simulink model "CRA_Assignment3"  (R2022b)
settings: Solver=VariableStepAuto  StartTime=0.0  StopTime=100  RelTol=1e-3
settings Model: Creator=lerio  LastModifiedBy=lerio

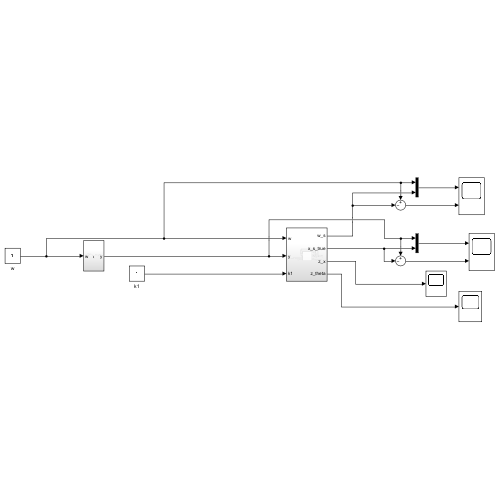
[thumbnail: Simulink's stored preview of the top-level diagram]
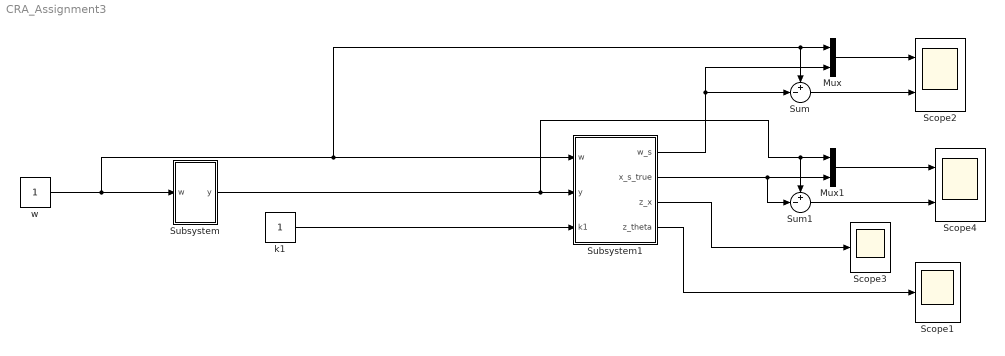
== system CRA_Assignment3 ==
  Mux : Mux  Inputs=2
  Mux1 : Mux  Inputs=2
  Scope1 : Scope
  Scope2 : Scope  NumInputPorts=2
  Scope3 : Scope
  Scope4 : Scope  NumInputPorts=2
  Subsystem : Subsystem
  Subsystem1 : Subsystem
  Sum : Sum  Inputs=+-|
  Sum1 : Sum  Inputs=+-|
  k1 : Constant
  w : Constant
  wires:
  w/1 -> Sum/1, Mux/1, Subsystem1/1(w), Subsystem/1(w)
  Subsystem/1(y) -> Sum1/1, Mux1/1, Subsystem1/2(y)
  k1/1 -> Subsystem1/3(k1)
  Mux/1 -> Scope2/1
  Subsystem1/1(w_s) -> Sum/2, Mux/2
  Sum/1 -> Scope2/2
  Mux1/1 -> Scope4/1
  Sum1/1 -> Scope4/2
  Subsystem1/2(x_s_true) -> Sum1/2, Mux1/2
  Subsystem1/3(z_x) -> Scope3/1
  Subsystem1/4(z_theta) -> Scope1/1

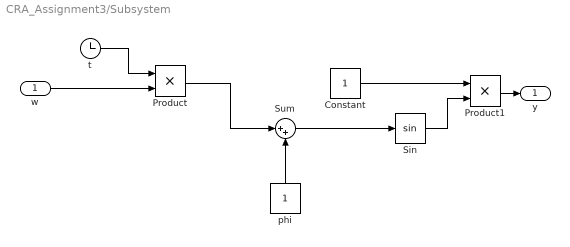
== system CRA_Assignment3/Subsystem ==
  w : Inport
  Constant : Constant
  Product : Product
  Product1 : Product
  Sin : Trigonometry
  Sum : Sum  Inputs=|++
  phi : Constant
  t : Clock
  y : Outport
  wires:
  Product1/1 -> y/1
  Constant/1 -> Product1/1
  Sin/1 -> Product1/2
  t/1 -> Product/1
  phi/1 -> Sum/2
  Product/1 -> Sum/1
  w/1 -> Product/2
  Sum/1 -> Sin/1

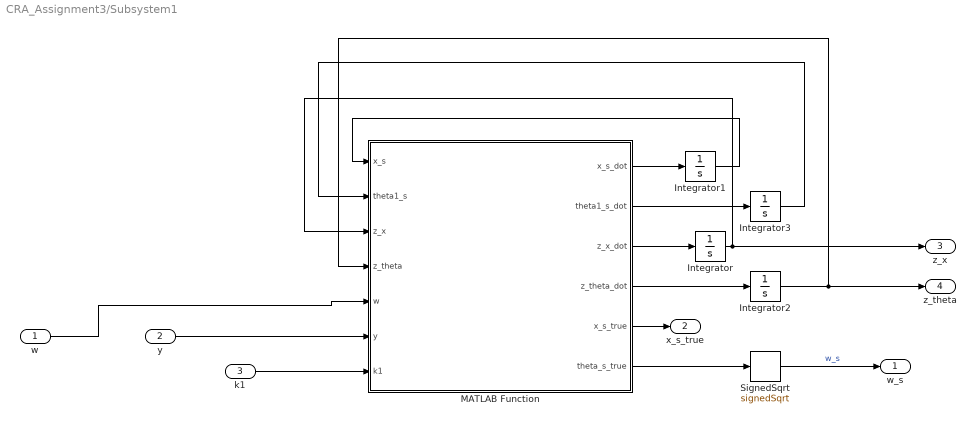
== system CRA_Assignment3/Subsystem1 ==
  w : Inport
  y : Inport  Port=2
  k1 : Inport  Port=3
  Integrator{,1..3} (4 alike) : Integrator
  MATLAB Function : MATLAB Function  TreatAsAtomicUnit=on
  SignedSqrt : Sqrt  Operator=signedSqrt  IntermediateResultsDataTypeStr=single
  w_s : Outport
  x_s_true : Outport  Port=2
  z_x : Outport  Port=3
  z_theta : Outport  Port=4
  wires:
  Integrator2/1 -> z_theta/1, MATLAB Function/4(z_theta)
  MATLAB Function/6(theta_s_true) -> SignedSqrt/1
  Integrator/1 -> z_x/1, MATLAB Function/3(z_x)
  MATLAB Function/1(x_s_dot) -> Integrator1/1
  Integrator3/1 -> MATLAB Function/2(theta1_s)
  MATLAB Function/4(z_theta_dot) -> Integrator2/1
  MATLAB Function/2(theta1_s_dot) -> Integrator3/1
  MATLAB Function/3(z_x_dot) -> Integrator/1
  Integrator1/1 -> MATLAB Function/1(x_s)
  MATLAB Function/5(x_s_true) -> x_s_true/1
  SignedSqrt/1 -> w_s/1  "w_s"
  y/1 -> MATLAB Function/6(y)
  k1/1 -> MATLAB Function/7(k1)
  w/1 -> MATLAB Function/5(w)

== matlab function CRA_Assignment3/Subsystem1/MATLAB Function ==
  data: x_s input; theta1_s input; z_x input; z_theta input; w input; y input; k1 input; x_s_dot output; theta1_s_dot output; z_x_dot output; z_theta_dot output; x_s_true output; theta_s_true output
function [x_s_dot, theta1_s_dot, z_x_dot, z_theta_dot, x_s_true, theta_s_true] = fcn(x_s, theta1_s, z_x, z_theta,w, y, k1)

theta1 = w^2;
delta = - x_s^2 * (y * x_s + theta1_s + k1^2) + y^2;
x_s_dot = -k1 * x_s - y;
theta1_s_dot = delta;

z_theta_dot = - x_s * z_x - (x_s^2) * z_theta - delta + theta1_s_dot;
z_x_dot = -k1 * z_x+(k1^2 + theta1)*(y + k1 * x_s + x_s_dot);

theta_s_true = y * x_s + theta1_s;
x_s_true = k1 * y + x_s*(k1^2 + theta1);
